simulink model "planar3dof_sim2a"  (R2017a)
settings: Solver=ode45  StartTime=0.0  StopTime=4  MaxStep=1e-2  RelTol=1e-3  EnableMultiTasking=on
values from neighbouring files (symbols this model uses):
  K = 1    [ex3.m]    (also in mdl_kinovagen3.m = 8.91; planar3dof.m = 50)
  q0 = [-pi/20 -pi/2]'    [ex3.m]    (also in planar3dof.m = [pi -pi/2 -pi/2])
libraries: dspmtrx3 x5, roblocks x3
settings Model: Creator=alexfneves  LastModifiedBy=rbp
settings DataIOCC: LimitDataPoints=on  SaveFormat=Array
settings OptimizationCC: LifeSpan=inf
settings DebuggingCC: SFUnexpectedBacktrackingDiag=warning  SFNoUnconditionalDefaultTransitionDiag=warning  SFExecutionAtInitializationDiag=none
settings HardwareCC: ProdBitPerPointer=32  ProdBitPerSizeT=32  ProdBitPerPtrDiffT=32  ProdLargestAtomicFloat=None  ProdIntDivRoundTo=Undefined  ProdEndianess=Unspecified  ProdWordSize=32  ProdHWDeviceType=32-bit Generic
settings ModelReferenceCC: PropagateSignalLabelsOutOfModel=off
settings GRTTargetCC: TargetLangStandard=C89/C90 (ANSI)  GeneratePreprocessorConditionals=Disable all
settings ConfigComp: CovMetricSettings=dw  CovHtmlReporting=on  CovSaveCumulativeToWorkspaceVar=on  CovSaveSingleToWorkspaceVar=on  CovExternalEMLEnable=off

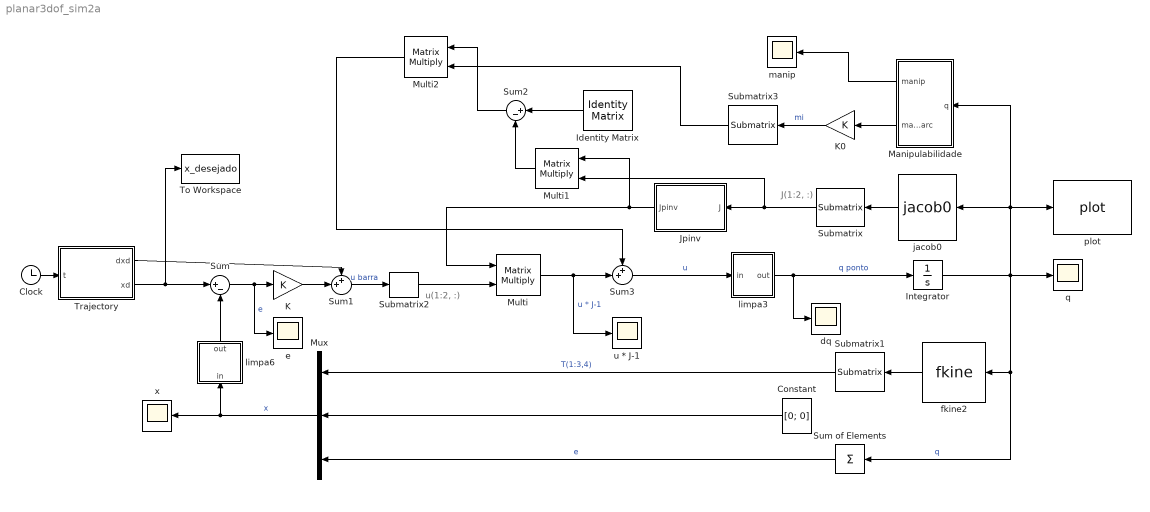
== system planar3dof_sim2a ==
  note: J(1:2, :)
  note: u(1:2, :)
  Clock : Clock
  Constant : Constant  Value=[0; 0]  VectorParams1D=off
  Identity Matrix : dspmtrx3/Identity Matrix  Inherit=off  N=3  Ts=1  dataType=double  isSigned=on  wordLen=16  udDataType=sfix(16)  fracBitsMode=Best precision  numFracBits=15  OutDataTypeStr=double  LastOutDataTypeStr=double
      settings: SourceProductName=DSP System Toolbox
  Integrator : Integrator  InitialCondition=q0
  Jpinv : MATLAB Function  TreatAsAtomicUnit=on
  K : Gain  Gain=K
  K0 : Gain  Gain=K
  Manipulabilidade : MATLAB Function  TreatAsAtomicUnit=on
  Multi : Product  Inputs=**  Multiplication=Matrix(*)
  Multi1 : Product  Inputs=**  Multiplication=Matrix(*)
  Multi2 : Product  Inputs=**  Multiplication=Matrix(*)
  Mux : Mux  Inputs=3
  Submatrix : dspmtrx3/Submatrix  RowSpan=Range of rows  RowStartMode=First  RowStartIndex=1  RowEndMode=Index  RowEndIndex=2  ColSpan=All columns  ColStartMode=First  ColStartIndex=1  ColEndMode=Index  ColEndIndex=3
  Submatrix1 : dspmtrx3/Submatrix  RowSpan=Range of rows  RowStartMode=First  RowStartIndex=1  RowEndMode=Offset from last  RowEndIndex=1  ColSpan=One column  ColStartMode=Last  ColStartIndex=1  ColEndMode=Last  ColEndIndex=1
  Submatrix2 : dspmtrx3/Submatrix  RowSpan=Range of rows  RowStartMode=First  RowStartIndex=1  RowEndMode=Index  RowEndIndex=2  ColSpan=All columns  ColStartMode=First  ColStartIndex=1  ColEndMode=Index  ColEndIndex=3
  Submatrix3 : dspmtrx3/Submatrix  RowSpan=Range of rows  RowStartMode=First  RowStartIndex=1  RowEndMode=Offset from last  RowEndIndex=0  ColSpan=One column  ColStartMode=Last  ColStartIndex=1  ColEndMode=Last  ColEndIndex=1
  Sum : Sum  Inputs=|+-
  Sum of Elements : Sum  Inputs=+
  Sum1 : Sum  Inputs=++|
  Sum2 : Sum  Inputs=|+-
  Sum3 : Sum  Inputs=++|
  To Workspace : ToWorkspace  VariableName=x_desejado  SaveFormat=Timeseries  SampleTime=-1
  Trajectory : MATLAB Function  TreatAsAtomicUnit=on
  dq : Scope
  e : Scope
  fkine2 : roblocks/Arm/fkine  robot=planar
  jacob0 : roblocks/Arm/jacob0   robot=planar
  limpa3 : MATLAB Function  TreatAsAtomicUnit=on
  limpa6 : MATLAB Function  TreatAsAtomicUnit=on
  manip : Scope
  plot : roblocks/Arm/plot  robot=planar  fps=5  holdplot=on
  q : Scope
  u * J-1 : Scope
  x : Scope
  wires:
  Sum/1 -> e/1, K/1  "e"
  Clock/1 -> Trajectory/1(t)
  fkine2/1 -> Submatrix1/1
  Mux/1 -> limpa6/1(in), x/1  "x"
  Trajectory/2(xd) -> To Workspace/1, Sum/1
  K/1 -> Sum1/2
  Trajectory/1(dxd) -> Sum1/1
  Submatrix1/1 -> Mux/1  "T(1:3,4)"
  Constant/1 -> Mux/2
  Sum3/1 -> limpa3/1(in)  "u"
  limpa6/1(out) -> Sum/2
  limpa3/1(out) -> dq/1, Integrator/1  "q ponto"
  Sum of Elements/1 -> Mux/3  "e"
  Integrator/1 -> q/1, plot/1, Manipulabilidade/1(q), jacob0/1, fkine2/1, Sum of Elements/1  "q"
  Manipulabilidade/1(manip) -> manip/1
  Manipulabilidade/2(manip_parc) -> K0/1
  jacob0/1 -> Submatrix/1
  Submatrix/1 -> Multi1/2, Jpinv/1(J)
  Identity Matrix/1 -> Sum2/1
  Multi1/1 -> Sum2/2
  Sum1/1 -> Submatrix2/1  "u barra"
  Submatrix2/1 -> Multi/2
  Jpinv/1(Jpinv) -> Multi1/1, Multi/1
  K0/1 -> Submatrix3/1  "mi"
  Multi/1 -> u * J-1/1, Sum3/2  "u * J-1"
  Multi2/1 -> Sum3/1
  Sum2/1 -> Multi2/1
  Submatrix3/1 -> Multi2/2

== matlab function planar3dof_sim2a/limpa6 ==
  data: out output; in input
function out = limpa(in)
%#codegen
    out = [in(1) in(2) in(3) in(4) in(5) in(6)]'
end

== matlab function planar3dof_sim2a/Trajectory ==
  data: dxd output; xd output; t input
function [dxd, xd] = trajectory(t)
%#codegen

    xd = xdFunc(t);
    dxd = dxdFunc(t);
end

== matlab function planar3dof_sim2a/limpa3 ==
  data: out output; in input
function out = limpa(in)
%#codegen
    out = [in(1) in(2) in(3)]'
end

== matlab function planar3dof_sim2a/Manipulabilidade ==
  data: q input; manip output; manip_parc output
function [manip, manip_parc] = Manip(q)
%#codegen

[manip, manip_parc] = manipFunc(q(1), q(2), q(3));

== matlab function planar3dof_sim2a/Jpinv ==
  data: J input; Jpinv output
function Jpinv = fcn(J)
%#codegen

Jpinv = pinv(J);
